simulink model "base_open_loop_model_compare"  (R2017a)
settings: Solver=ode45  StartTime=0.0  StopTime=2  FixedStep=0.01  RelTol=1e-3  EnableMultiTasking=on
settings Model: Creator=cpmcclel  LastModifiedBy=s6bae
settings DataIOCC: LimitDataPoints=on  SaveFormat=Array
settings OptimizationCC: LifeSpan=inf
settings DebuggingCC: SolverPrmCheckMsg=warning  SFUnexpectedBacktrackingDiag=warning  SFNoUnconditionalDefaultTransitionDiag=warning  SFExecutionAtInitializationDiag=none
settings HardwareCC: ProdBitPerPointer=32  ProdBitPerSizeT=32  ProdBitPerPtrDiffT=32  ProdLargestAtomicFloat=None  ProdIntDivRoundTo=Undefined  ProdEndianess=Unspecified  ProdWordSize=32  ProdHWDeviceType=32-bit Generic
settings ModelReferenceCC: PropagateSignalLabelsOutOfModel=off
settings GRTTargetCC: TargetLangStandard=C89/C90 (ANSI)  GeneratePreprocessorConditionals=Disable all
settings ConfigComp: CovMetricSettings=dw  CovHtmlReporting=on  CovSaveCumulativeToWorkspaceVar=on  CovSaveSingleToWorkspaceVar=on  CovExternalEMLEnable=off  CovSFcnEnable=off

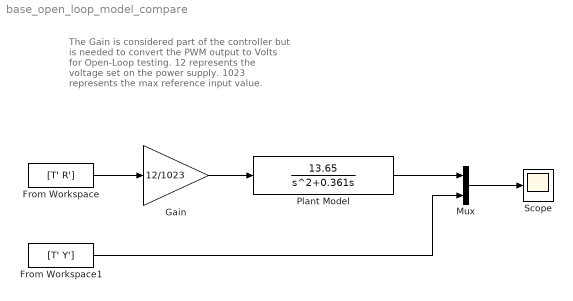
== system base_open_loop_model_compare ==
  note: The Gain is considered part of the controller but is needed to convert the PWM output to Volts for Open-Loop testing. 12 represents the voltage set on the power supply. 1023 represents the max reference input value.
  From Workspace : FromWorkspace  VariableName=[T' R']  SampleTime=.01
  From Workspace1 : FromWorkspace  VariableName=[T' Y']
  Gain : Gain  Gain=12/1023
  Mux : Mux  Inputs=2
  Plant Model : TransferFcn  Numerator=[13.65]  Denominator=[1 0.361 0]
  Scope : Scope
  wires:
  Mux/1 -> Scope/1
  From Workspace1/1 -> Mux/2
  Plant Model/1 -> Mux/1
  Gain/1 -> Plant Model/1
  From Workspace/1 -> Gain/1
